simulink model "gm_HDL_pfc_gold_fi_vnl"  (R2024b)
settings: Solver=FixedStepDiscrete  StartTime=0.0  StopTime=.06  RelTol=1e-3
InitFcn:
  | fidelity_pfc_vals;
  | load('C:\Users\angro\Desktop\hil\pfc3ph\matlab\sim\sschdl\pfc_desktop\stateSpaceParameters.mat');
undefined symbols (not defined in the file or in its folder): a, b, c, DiscIntNeverNeededParam, fsw, Gs, s, stateSpaceParameters_1, t_ss, tsw
libraries: simulink x55, hdlmdlgenlib x26, hdlsllib x10, mcbcontrolslib x5, dspsrcs4 x3, slpidlib x2, hdlssclib x2, spsSVPWMGenerator2LevelLib x1, spsPLL3phLib x1
(part 2 of 4)

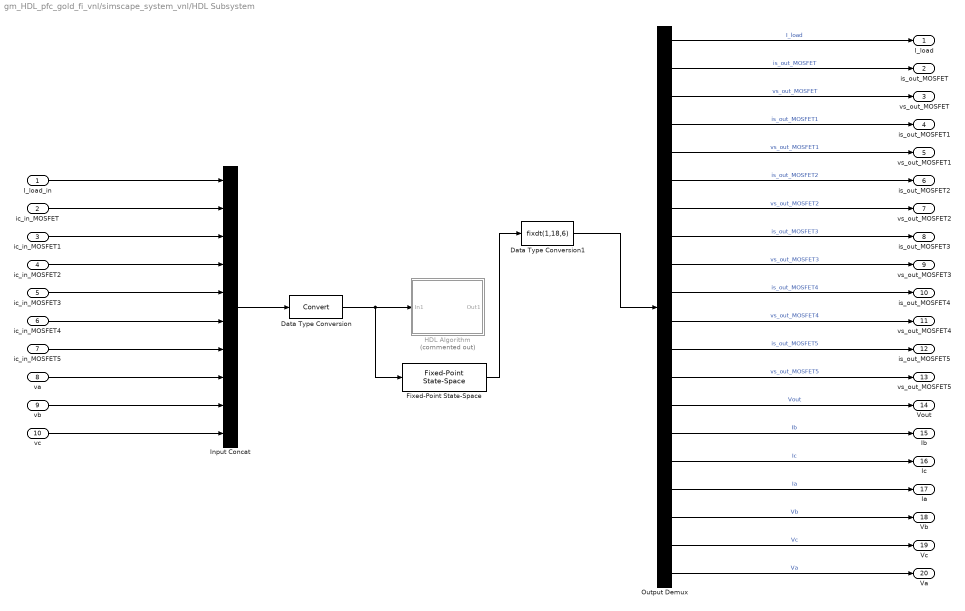
== system gm_HDL_pfc_gold_fi_vnl/simscape_system_vnl/HDL Subsystem ==
  I_load_in : Inport  OutDataTypeStr=fixdt(1,18,8)
  ic_in_MOSFET : Inport  Port=2  OutDataTypeStr=fixdt(1,18,8)
  ic_in_MOSFET1 : Inport  Port=3  OutDataTypeStr=fixdt(1,18,8)
  ic_in_MOSFET2 : Inport  Port=4  OutDataTypeStr=fixdt(1,18,8)
  ic_in_MOSFET3 : Inport  Port=5  OutDataTypeStr=fixdt(1,18,8)
  ic_in_MOSFET4 : Inport  Port=6  OutDataTypeStr=fixdt(1,18,8)
  ic_in_MOSFET5 : Inport  Port=7  OutDataTypeStr=fixdt(1,18,8)
  va : Inport  Port=8  OutDataTypeStr=fixdt(1,18,8)
  vb : Inport  Port=9  OutDataTypeStr=fixdt(1,18,8)
  vc : Inport  Port=10  OutDataTypeStr=fixdt(1,18,8)
  Data Type Conversion : DataTypeConversion  SaturateOnIntegerOverflow=off  RndMeth=Floor
  Data Type Conversion1 : DataTypeConversion  OutDataTypeStr=fixdt(1,18,6)  SaturateOnIntegerOverflow=off  RndMeth=Floor
  Fixed-Point State-Space : simulink/Additional Math & Discrete/Additional Discrete/Fixed-Point State-Space  A=fi(stateSpaceParameters_1.Ad,1,25,24)  B=fi(stateSpaceParameters_1.Bd,1,25,31)  C=fi(stateSpaceParameters_1.Cd,1,25,20)  D=fi(stateSpaceParameters_1.Dd,1,25,19)  InitialCondition=fi(stateSpaceParameters_1.X0,1,25,14)  InternalDataType=fixdt(1,25,13)  StateEqScaling=2^0  OutputEqScaling=2^0  DoSatur=off
  HDL Algorithm : Subsystem  Commented=on
  Input Concat : Concatenate  NumInputs=10
  Output Demux : Demux  Outputs=20
  I_load : Outport
  is_out_MOSFET : Outport  Port=2
  vs_out_MOSFET : Outport  Port=3
  is_out_MOSFET1 : Outport  Port=4
  vs_out_MOSFET1 : Outport  Port=5
  is_out_MOSFET2 : Outport  Port=6
  vs_out_MOSFET2 : Outport  Port=7
  is_out_MOSFET3 : Outport  Port=8
  vs_out_MOSFET3 : Outport  Port=9
  is_out_MOSFET4 : Outport  Port=10
  vs_out_MOSFET4 : Outport  Port=11
  is_out_MOSFET5 : Outport  Port=12
  vs_out_MOSFET5 : Outport  Port=13
  Vout : Outport  Port=14
  Ib : Outport  Port=15
  Ic : Outport  Port=16
  Ia : Outport  Port=17
  Vb : Outport  Port=18
  Vc : Outport  Port=19
  Va : Outport  Port=20
  wires:
  Fixed-Point State-Space/1 -> Data Type Conversion1/1
  Data Type Conversion/1 -> HDL Algorithm/1(In1), Fixed-Point State-Space/1
  Data Type Conversion1/1 -> Output Demux/1
  ic_in_MOSFET4/1 -> Input Concat/6
  va/1 -> Input Concat/8
  ic_in_MOSFET5/1 -> Input Concat/7
  ic_in_MOSFET2/1 -> Input Concat/4
  ic_in_MOSFET3/1 -> Input Concat/5
  I_load_in/1 -> Input Concat/1
  ic_in_MOSFET1/1 -> Input Concat/3
  vb/1 -> Input Concat/9
  Output Demux/20 -> Va/1  "Va"
  Output Demux/18 -> Vb/1  "Vb"
  Output Demux/19 -> Vc/1  "Vc"
  Output Demux/16 -> Ic/1  "Ic"
  Output Demux/14 -> Vout/1  "Vout"
  Output Demux/11 -> vs_out_MOSFET4/1  "vs_out_MOSFET4"
  Output Demux/9 -> vs_out_MOSFET3/1  "vs_out_MOSFET3"
  Output Demux/10 -> is_out_MOSFET4/1  "is_out_MOSFET4"
  Output Demux/12 -> is_out_MOSFET5/1  "is_out_MOSFET5"
  Output Demux/5 -> vs_out_MOSFET1/1  "vs_out_MOSFET1"
  Output Demux/13 -> vs_out_MOSFET5/1  "vs_out_MOSFET5"
  Output Demux/15 -> Ib/1  "Ib"
  Output Demux/8 -> is_out_MOSFET3/1  "is_out_MOSFET3"
  Output Demux/6 -> is_out_MOSFET2/1  "is_out_MOSFET2"
  vc/1 -> Input Concat/10
  Output Demux/1 -> I_load/1  "I_load"
  Output Demux/17 -> Ia/1  "Ia"
  Input Concat/1 -> Data Type Conversion/1
  ic_in_MOSFET/1 -> Input Concat/2
  Output Demux/4 -> is_out_MOSFET1/1  "is_out_MOSFET1"
  Output Demux/3 -> vs_out_MOSFET/1  "vs_out_MOSFET"
  Output Demux/2 -> is_out_MOSFET/1  "is_out_MOSFET"
  Output Demux/7 -> vs_out_MOSFET2/1  "vs_out_MOSFET2"

== system gm_HDL_pfc_gold_fi_vnl/Subsystem1/ctrl_pwm/PI_CTRL ==
  id : Inport
  iq : Inport  Port=2
  Add3 : Sum  Inputs=+-
  Add4 : Sum  Inputs=+-
  Constant : Constant  Value=0  SampleTime=t_ss
  Constant1 : Constant  Value=-6  SampleTime=t_ss
  Vd_ctrl : slpidlib/PID Controller  Controller=PI  Form=Parallel  TimeDomain=Discrete-time  UseExternalTs=off  SampleTime=t_ss  IntegratorMethod=Backward Euler  FilterMethod=Forward Euler  ControllerParametersSource=internal  P=-1.8  I=-.15  UseKiTs=off  D=0  UseExternalDerivativeSource=off  N=100  UseFilter=on  TunerSelectOption=Transfer Function Based (PID Tuner App)  InitialConditionSource=internal  InitialConditionForIntegrator=0  InitialConditionForFilter=0  DifferentiatorICPrevScaledInput=0  ExternalReset=none  TrackingMode=off  Kt=1  LimitOutput=off  SatLimitsSource=internal  UpperSaturationLimit=5e2  LowerSaturationLimit=-5e2  LinearizeAsGain=on  AntiWindupMode=clamping  Kb=1  LimitIntegrator=off  UpperIntegratorSaturationLimit=inf  LowerIntegratorSaturationLimit=-inf  POutMin=[]  POutMax=[]  IOutMin=[]  IOutMax=[]  DOutMin=[]  DOutMax=[]  NOutMin=[]  NOutMax=[]  SumOutMin=[]  SumOutMax=[]  SaturationOutMin=[]  SaturationOutMax=[]  PParamMin=[]  PParamMax=[]  IParamMin=[]  IParamMax=[]  DParamMin=[]  DParamMax=[]  NParamMin=[]  NParamMax=[]  KbParamMin=[]  KbParamMax=[]  KtParamMin=[]  KtParamMax=[]  KbOutMin=[]  KbOutMax=[]  KtOutMin=[]  KtOutMax=[]  IntegratorOutMin=[]  IntegratorOutMax=[]  FilterOutMin=[]  FilterOutMax=[]  SumI1OutMin=[]  SumI1OutMax=[]  SumI2OutMin=[]  SumI2OutMax=[]  SumI3OutMin=[]  SumI3OutMax=[]  SumI4OutMin=[]  SumI4OutMax=[]  SumDOutMin=[]  SumDOutMax=[]  DifferentiatorOutMin=[]  DifferentiatorOutMax=[]  FilterDiffOutCoefMin=[]  FilterDiffOutCoefMax=[]  ReciprocalOutMin=[]  ReciprocalOutMax=[]  SumDenOutMin=[]  SumDenOutMax=[]  SumNumOutMin=[]  SumNumOutMax=[]  DivideOutMin=[]  DivideOutMax=[]  UdiffTsProdOutMin=[]  UdiffTsProdOutMax=[]  NTsProdOutMin=[]  NTsProdOutMax=[]  UintegralTsProdOutMin=[]  UintegralTsProdOutMax=[]  UngainTsProdOutMin=[]  UngainTsProdOutMax=[]  ClampingZeroOutDataTypeStr=Inherit: Inherit via back propagation  ClampingZeroOutMin=[]  ClampingZeroOutMax=[]  FilterDenConstantOutDataTypeStr=Inherit: Inherit via back propagation  FilterDenConstantOutMin=[]  FilterDenConstantOutMax=[]  PCopyOutDataTypeStr=Inherit: Inherit via back propagation  PCopyOutMin=[]  PCopyOutMax=[]  NCopyOutDataTypeStr=Inherit: Inherit via back propagation  NCopyOutMin=[]  NCopyOutMax=[]  IntegratorContinuousStateAttributes=''  IntegratorStateMustResolveToSignalObject=off  IntegratorRTWStateStorageClass=Auto  FilterContinuousStateAttributes=''  FilterStateMustResolveToSignalObject=off  FilterRTWStateStorageClass=Auto  ParallelPVariant=InternalParameters  IdealPVariant=Disabled  IVariant=InternalParameters  DVariant=Disabled  IntegratorVariant=Discrete  SatVariant=Disabled  AWVariant=Passthrough  PCopyVariant=Disabled  TRVariant=Disabled  FdbkBlocksVariant=Forward  IdealPFdbkVariant=Disabled  SatFdbkVariant=Disabled  DerivativeFilterVariant=Disabled  NVariant=Disabled  NCopyVariant=Disabled_SignalSpec  FilterICVariant=Disabled  IntegratorICVariant=InternalICs  ExternalResetVariant=Disabled  TRSumVariant=Passthrough  SumFdbkVariant=Disabled  SumVariant=Sum_PI  TsampFilterVariant=InternalTs  TsampNgainVariant=Passthrough  TsampIntegralVariant=Disabled_SignalSpec  ExternalSaturationOutDataTypeStr=Inherit: Same as second input  DerivativeSourceVariant=Disabled  PreIntVariant=InternalPreInt
  Vq_ctrl : slpidlib/PID Controller  Controller=PI  Form=Parallel  TimeDomain=Discrete-time  UseExternalTs=off  SampleTime=t_ss  IntegratorMethod=Backward Euler  FilterMethod=Forward Euler  ControllerParametersSource=internal  P=-2  I=-.2  UseKiTs=off  D=0  UseExternalDerivativeSource=off  N=100  UseFilter=on  TunerSelectOption=Transfer Function Based (PID Tuner App)  InitialConditionSource=internal  InitialConditionForIntegrator=0  InitialConditionForFilter=0  DifferentiatorICPrevScaledInput=0  ExternalReset=none  TrackingMode=off  Kt=1  LimitOutput=off  SatLimitsSource=internal  UpperSaturationLimit=5e2  LowerSaturationLimit=-5e2  LinearizeAsGain=on  AntiWindupMode=clamping  Kb=1  LimitIntegrator=off  UpperIntegratorSaturationLimit=inf  LowerIntegratorSaturationLimit=-inf  POutMin=[]  POutMax=[]  IOutMin=[]  IOutMax=[]  DOutMin=[]  DOutMax=[]  NOutMin=[]  NOutMax=[]  SumOutMin=[]  SumOutMax=[]  SaturationOutMin=[]  SaturationOutMax=[]  PParamMin=[]  PParamMax=[]  IParamMin=[]  IParamMax=[]  DParamMin=[]  DParamMax=[]  NParamMin=[]  NParamMax=[]  KbParamMin=[]  KbParamMax=[]  KtParamMin=[]  KtParamMax=[]  KbOutMin=[]  KbOutMax=[]  KtOutMin=[]  KtOutMax=[]  IntegratorOutMin=[]  IntegratorOutMax=[]  FilterOutMin=[]  FilterOutMax=[]  SumI1OutMin=[]  SumI1OutMax=[]  SumI2OutMin=[]  SumI2OutMax=[]  SumI3OutMin=[]  SumI3OutMax=[]  SumI4OutMin=[]  SumI4OutMax=[]  SumDOutMin=[]  SumDOutMax=[]  DifferentiatorOutMin=[]  DifferentiatorOutMax=[]  FilterDiffOutCoefMin=[]  FilterDiffOutCoefMax=[]  ReciprocalOutMin=[]  ReciprocalOutMax=[]  SumDenOutMin=[]  SumDenOutMax=[]  SumNumOutMin=[]  SumNumOutMax=[]  DivideOutMin=[]  DivideOutMax=[]  UdiffTsProdOutMin=[]  UdiffTsProdOutMax=[]  NTsProdOutMin=[]  NTsProdOutMax=[]  UintegralTsProdOutMin=[]  UintegralTsProdOutMax=[]  UngainTsProdOutMin=[]  UngainTsProdOutMax=[]  ClampingZeroOutDataTypeStr=Inherit: Inherit via back propagation  ClampingZeroOutMin=[]  ClampingZeroOutMax=[]  FilterDenConstantOutDataTypeStr=Inherit: Inherit via back propagation  FilterDenConstantOutMin=[]  FilterDenConstantOutMax=[]  PCopyOutDataTypeStr=Inherit: Inherit via back propagation  PCopyOutMin=[]  PCopyOutMax=[]  NCopyOutDataTypeStr=Inherit: Inherit via back propagation  NCopyOutMin=[]  NCopyOutMax=[]  IntegratorContinuousStateAttributes=''  IntegratorStateMustResolveToSignalObject=off  IntegratorRTWStateStorageClass=Auto  FilterContinuousStateAttributes=''  FilterStateMustResolveToSignalObject=off  FilterRTWStateStorageClass=Auto  ParallelPVariant=InternalParameters  IdealPVariant=Disabled  IVariant=InternalParameters  DVariant=Disabled  IntegratorVariant=Discrete  SatVariant=Disabled  AWVariant=Passthrough  PCopyVariant=Disabled  TRVariant=Disabled  FdbkBlocksVariant=Forward  IdealPFdbkVariant=Disabled  SatFdbkVariant=Disabled  DerivativeFilterVariant=Disabled  NVariant=Disabled  NCopyVariant=Disabled_SignalSpec  FilterICVariant=Disabled  IntegratorICVariant=InternalICs  ExternalResetVariant=Disabled  TRSumVariant=Passthrough  SumFdbkVariant=Disabled  SumVariant=Sum_PI  TsampFilterVariant=InternalTs  TsampNgainVariant=Passthrough  TsampIntegralVariant=Disabled_SignalSpec  ExternalSaturationOutDataTypeStr=Inherit: Same as second input  DerivativeSourceVariant=Disabled  PreIntVariant=InternalPreInt
  Vd_inductor : Outport
  Vq_inductor : Outport  Port=2
  wires:
  Add3/1 -> Vd_ctrl/1  "error_id"
  id/1 -> Add3/2
  Constant/1 -> Add3/1
  iq/1 -> Add4/2
  Add4/1 -> Vq_ctrl/1  "error_iq"
  Vd_ctrl/1 -> Vd_inductor/1
  Vq_ctrl/1 -> Vq_inductor/1
  Constant1/1 -> Add4/1

== system gm_HDL_pfc_gold_fi_vnl/Subsystem1/ctrl_pwm/SVPWM ==
  Vd_inductor : Inport
  angle : Inport  Port=2
  Vq_inductor : Inport  Port=3
  Cos : Trigonometry  Operator=cos
  Inverse Park Transform : mcbcontrolslib/Inverse Park Transform  PhaseInput=Two inputs  AxisAlignment=D-axis  ThetaInput=Sine and Cosine electrical position  AngleInput=Per-unit  N_points=1024
  SVPWM Generator (2-Level) : spsSVPWMGenerator2LevelLib/SVPWM Generator (2-Level)  InputType=alpha-beta components  SwitchingPattern=Pattern #1  Fc=fsw*1e3  ParUref=[0.8 -30 50]  Ts=t_ss
  Sin : Trigonometry
  P : Outport
  wires:
  Vd_inductor/1 -> Inverse Park Transform/1
  Vq_inductor/1 -> Inverse Park Transform/2
  Inverse Park Transform/2 -> SVPWM Generator (2-Level)/2  "Vbet_indc"
  Sin/1 -> Inverse Park Transform/3
  Cos/1 -> Inverse Park Transform/4
  Inverse Park Transform/1 -> SVPWM Generator (2-Level)/1  "Valp_indc"
  angle/1 -> Cos/1, Sin/1
  SVPWM Generator (2-Level)/1 -> P/1

== system gm_HDL_pfc_gold_fi_vnl/Subsystem1/ctrl_pwm/transforms ==
  a : Inport
  b : Inport  Port=2
  In3 : Inport  Port=3
  In4 : Inport  Port=4
  In5 : Inport  Port=5
  Claro-Parl Transform : Subsystem  Commented=on
  Claro-Parl Transform1 : Subsystem
  Delay : Delay  DelayLength=1
  Delay1 : Delay  DelayLength=1
  Mux : Mux  Inputs=3
  PLL (3ph) : spsPLL3phLib/PLL (3ph)  Fmin=50  Par_Init=[0, 50]  ParK=[180,3200,1]  TcD=1e-4  MaxRateChangeFreq=12  FilterCutOffFreq=25  Ts=t_ss  AGC=on
  Terminator : Terminator
  id : Outport
  iq : Outport  Port=2
  angle : Outport  Port=3
  wires:
  Mux/1 -> PLL (3ph)/1
  PLL (3ph)/2 -> angle/1, Claro-Parl Transform1/3(wt), Claro-Parl Transform/3(wt)  "angle"
  PLL (3ph)/1 -> Terminator/1
  In3/1 -> Mux/1, Claro-Parl Transform/1(a)
  In5/1 -> Mux/3
  b/1 -> Delay1/1
  In4/1 -> Claro-Parl Transform/2(b), Mux/2
  a/1 -> Delay/1
  Delay/1 -> Claro-Parl Transform1/1(a)
  Delay1/1 -> Claro-Parl Transform1/2(b)
  Claro-Parl Transform/1(d) -> ?  "vd"
  Claro-Parl Transform/2(q) -> ?  "vq"
  Claro-Parl Transform1/1(d) -> id/1  "id"
  Claro-Parl Transform1/2(q) -> iq/1  "iq"

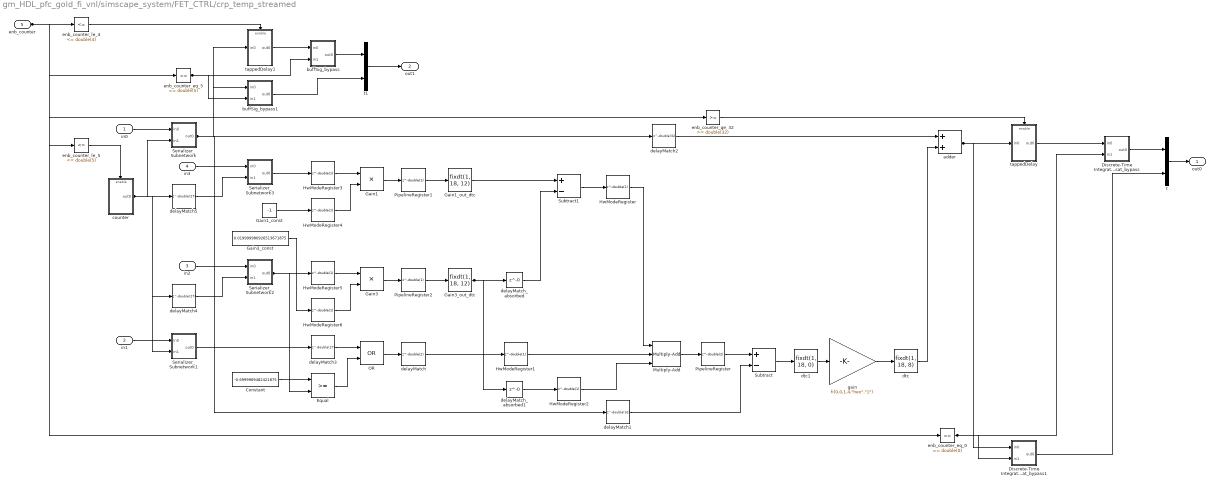
== system gm_HDL_pfc_gold_fi_vnl/simscape_system/FET_CTRL/crp_temp_streamed ==
  in0 : Inport  OutDataTypeStr=fixdt(1, 18, 8)  PortDimensions=[6]  SampleTime=1.38600138600139e-08
  in1 : Inport  Port=2  OutDataTypeStr=boolean  PortDimensions=[6]  SampleTime=1.38600138600139e-08
  in2 : Inport  Port=3  OutDataTypeStr=fixdt(1, 18, 6)  PortDimensions=[6]  SampleTime=1.38600138600139e-08
  in3 : Inport  Port=4  OutDataTypeStr=fixdt(1, 18, 6)  PortDimensions=[6]  SampleTime=1.38600138600139e-08
  enb_counter : Inport  Port=5  OutDataTypeStr=fixdt(0, 6, 0)  SampleTime=1.38600138600139e-08
  Constant : Constant  Value=-0.6999969482421875  OutDataTypeStr=fixdt(1, 18, 17)  SampleTime=1.38600138600139e-08
  Discrete-Time Integrator_u_sat_bypass : Subsystem
  Discrete-Time Integrator_u_sat_bypass1 : Subsystem
  Equal : RelationalOperator  OutDataTypeStr=boolean  SampleTime=1.38600138600139e-08  InputSameDT=off
  Gain1 : Product  Inputs=**  OutDataTypeStr=fixdt(1, 36, 23)  SampleTime=1.38600138600139e-08
  Gain1_const : Constant  Value=-1  OutDataTypeStr=fixdt(1, 18, 17)  SampleTime=1.38600138600139e-08
  Gain1_out_dtc : DataTypeConversion  OutDataTypeStr=fixdt(1, 18, 12)  SampleTime=1.38600138600139e-08  SaturateOnIntegerOverflow=off  RndMeth=Floor
  Gain3 : Product  Inputs=**  OutDataTypeStr=fixdt(1, 36, 28)  SampleTime=1.38600138600139e-08
  Gain3_const : Constant  Value=0.019999980926513671875  OutDataTypeStr=fixdt(1, 18, 22)  SampleTime=1.38600138600139e-08
  Gain3_out_dtc : DataTypeConversion  OutDataTypeStr=fixdt(1, 18, 12)  SampleTime=1.38600138600139e-08  SaturateOnIntegerOverflow=off  RndMeth=Floor
  HwModeRegister{,1..6} (7 alike) : Delay  DelayLength=double(1)  InitialCondition=0  SampleTime=1.38600138600139e-08
  Multiply-Add : hdlsllib/HDL Operations/Multiply-Add  Function=c+(a.*b)  datatype=fixdt(1, 18, 12)  DoSatur=off  FMA=off
  OR : Logic  Operator=OR  AllPortsSameDT=off  OutDataTypeStr=boolean  SampleTime=1.38600138600139e-08
  PipelineRegister : Delay  DelayLength=double(2)  InitialCondition=0  SampleTime=1.38600138600139e-08
  PipelineRegister1 : Delay  DelayLength=double(1)  InitialCondition=0  SampleTime=1.38600138600139e-08
  PipelineRegister2 : Delay  DelayLength=double(1)  InitialCondition=0  SampleTime=1.38600138600139e-08
  Serializer_Subnetwork : Subsystem
  Serializer_Subnetwork1 : Subsystem
  Serializer_Subnetwork2 : Subsystem
  Serializer_Subnetwork3 : Subsystem
  Subtract : Sum  Inputs=+-  OutDataTypeStr=fixdt(1, 18, 12)  AccumDataTypeStr=fixdt(1, 23, 12)  SampleTime=1.38600138600139e-08
  Subtract1 : Sum  Inputs=+-  OutDataTypeStr=fixdt(1, 18, 11)  AccumDataTypeStr=fixdt(1, 19, 12)  SampleTime=1.38600138600139e-08
  adder : Sum  OutDataTypeStr=fixdt(1, 18, 8)  AccumDataTypeStr=fixdt(1, 18, 8)  SampleTime=1.38600138600139e-08
  buffSig_bypass : Subsystem
  buffSig_bypass1 : Subsystem
  counter : Subsystem
  delayMatch : Delay  DelayLength=double(2)  InitialCondition=0  SampleTime=1.38600138600139e-08
  delayMatch1 : Delay  DelayLength=double(32)  InitialCondition=0  SampleTime=1.38600138600139e-08
  delayMatch2 : Delay  DelayLength=double(32)  InitialCondition=0  SampleTime=1.38600138600139e-08
  delayMatch3 : Delay  DelayLength=double(27)  InitialCondition=0  SampleTime=1.38600138600139e-08
  delayMatch4 : Delay  DelayLength=double(27)  InitialCondition=0  SampleTime=1.38600138600139e-08
  delayMatch5 : Delay  DelayLength=double(27)  InitialCondition=0  SampleTime=1.38600138600139e-08
  delayMatch_absorbed : Delay  DelayLength=0
  delayMatch_absorbed1 : Delay  DelayLength=0
  dtc : DataTypeConversion  OutDataTypeStr=fixdt(1, 18, 8)  ConvertRealWorld=Stored Integer (SI)  SampleTime=1.38600138600139e-08  SaturateOnIntegerOverflow=off  RndMeth=Floor
  dtc1 : DataTypeConversion  OutDataTypeStr=fixdt(1, 18, 0)  ConvertRealWorld=Stored Integer (SI)  SampleTime=1.38600138600139e-08  SaturateOnIntegerOverflow=off  RndMeth=Floor
  enb_counter_eq_0 : simulink/Logic and Bit Operations/Compare To Constant  relop===  const=double(0)  OutDataTypeStr=boolean
  enb_counter_eq_5 : simulink/Logic and Bit Operations/Compare To Constant  relop===  const=double(5)  OutDataTypeStr=boolean
  enb_counter_ge_32 : simulink/Logic and Bit Operations/Compare To Constant  relop=>=  const=double(32)  OutDataTypeStr=boolean
  enb_counter_le_4 : simulink/Logic and Bit Operations/Compare To Constant  relop=<=  const=double(4)  OutDataTypeStr=boolean
  enb_counter_le_5 : simulink/Logic and Bit Operations/Compare To Constant  relop=<=  const=double(5)  OutDataTypeStr=boolean
  gain : Gain  Gain="fi(0,0,1,4,\"hex\",\"1\")"  ParamDataTypeStr=fixdt(0, 1, 4)  OutDataTypeStr=fixdt(1, 18, 0)  SampleTime=1.38600138600139e-08
  t : Mux  Inputs=2
  t1 : Mux  Inputs=2
  tappedDelay : Subsystem
  tappedDelay1 : Subsystem
  out0 : Outport  OutDataTypeStr=fixdt(1, 18, 8)  PortDimensions=[6]  SampleTime=1.38600138600139e-08
  out1 : Outport  Port=2  OutDataTypeStr=fixdt(1, 18, 8)  PortDimensions=[6]  SampleTime=1.38600138600139e-08
  wires:
  Discrete-Time Integrator_u_sat_bypass/1(out0) -> t/1
  enb_counter_eq_0/1 -> Discrete-Time Integrator_u_sat_bypass1/2(in1), Discrete-Time Integrator_u_sat_bypass/2(in1)
  adder/1 -> Discrete-Time Integrator_u_sat_bypass1/1(in0), tappedDelay/1(in0)
  dtc/1 -> adder/2
  gain/1 -> dtc/1
  dtc1/1 -> gain/1
  Subtract/1 -> dtc1/1
  PipelineRegister/1 -> Subtract/1
  enb_counter_ge_32/1 -> tappedDelay/Enable
  Multiply-Add/1 -> PipelineRegister/1
  delayMatch1/1 -> Subtract/2
  delayMatch_absorbed1/1 -> HwModeRegister2/1
  delayMatch_absorbed/1 -> Subtract1/2
  Gain1_out_dtc/1 -> Subtract1/1
  PipelineRegister1/1 -> Gain1_out_dtc/1
  OR/1 -> delayMatch/1
  Gain3/1 -> PipelineRegister2/1
  Gain1/1 -> PipelineRegister1/1
  t1/1 -> out1/1
  delayMatch/1 -> HwModeRegister1/1
  Equal/1 -> OR/2
  HwModeRegister/1 -> Multiply-Add/1
  HwModeRegister6/1 -> Gain3/2
  HwModeRegister5/1 -> Gain3/1
  HwModeRegister4/1 -> Gain1/2
  HwModeRegister3/1 -> Gain1/1
  delayMatch3/1 -> OR/1
  Constant/1 -> Equal/1
  Gain3_out_dtc/1 -> delayMatch_absorbed1/1, delayMatch_absorbed/1
  Serializer_Subnetwork2/1(out0) -> HwModeRegister5/1, Equal/2
  Gain1_const/1 -> HwModeRegister4/1
  buffSig_bypass1/1(out0) -> t1/2
  tappedDelay1/1(out0) -> buffSig_bypass/1(in0)
  PipelineRegister2/1 -> Gain3_out_dtc/1
  delayMatch4/1 -> Serializer_Subnetwork2/2(in1)
  Discrete-Time Integrator_u_sat_bypass1/1(out0) -> t/2
  in2/1 -> Serializer_Subnetwork2/1(in0)
  delayMatch2/1 -> adder/1
  delayMatch5/1 -> Serializer_Subnetwork3/2(in1)
  HwModeRegister2/1 -> Multiply-Add/3
  in3/1 -> Serializer_Subnetwork3/1(in0)
  t/1 -> out0/1
  Serializer_Subnetwork/1(out0) -> buffSig_bypass1/1(in0), delayMatch1/1, delayMatch2/1, tappedDelay1/1(in0)
  in1/1 -> Serializer_Subnetwork1/1(in0)
  buffSig_bypass/1(out0) -> t1/1
  HwModeRegister1/1 -> Multiply-Add/2
  counter/1(out0) -> Serializer_Subnetwork/2(in1), Serializer_Subnetwork1/2(in1), delayMatch4/1, delayMatch5/1
  Serializer_Subnetwork3/1(out0) -> HwModeRegister3/1
  in0/1 -> Serializer_Subnetwork/1(in0)
  enb_counter_le_4/1 -> tappedDelay1/Enable
  enb_counter_le_5/1 -> counter/Enable
  Serializer_Subnetwork1/1(out0) -> delayMatch3/1
  Gain3_const/1 -> HwModeRegister6/1
  enb_counter_eq_5/1 -> buffSig_bypass1/2(in1), buffSig_bypass/2(in1)
  Subtract1/1 -> HwModeRegister/1
  enb_counter/1 -> enb_counter_le_4/1, enb_counter_le_5/1, enb_counter_eq_0/1, enb_counter_eq_5/1, enb_counter_ge_32/1
  tappedDelay/1(out0) -> Discrete-Time Integrator_u_sat_bypass/1(in0)

== system gm_HDL_pfc_gold_fi_vnl/simscape_system/HDL Subsystem/Sparse Matrix-Vector Product ==
  in0 : Inport  OutDataTypeStr=fixdt(1, 25, 13)  PortDimensions=[10]  SampleTime=1.38600138600139e-08
  selectSignal : Inport  Port=2  OutDataTypeStr=boolean  SampleTime=1.38600138600139e-08
  enb_counter : Inport  Port=3  OutDataTypeStr=fixdt(0, 6, 0)  SampleTime=1.38600138600139e-08
  SelectCols{1..6} (6 alike) : Selector  InputPortWidth=10  IndexOptions=Index vector (dialog)  Indices=double([2 3 4 5 6 7 8 9 10])  OutputSizes=double(1)
  SelectCols7 : Selector  InputPortWidth=10  IndexOptions=Index vector (dialog)  Indices=double([1 2 3 4 5 6 7 8 9])  OutputSizes=double(1)
  SelectRows1 : Selector  InputPortWidth=63  IndexOptions=Index vector (dialog)  Indices=double([2 9 16 23 30 37 44 51 58])  OutputSizes=double(1)
  SelectRows2 : Selector  InputPortWidth=63  IndexOptions=Index vector (dialog)  Indices=double([3 10 17 24 31 38 45 52 59])  OutputSizes=double(1)
  SelectRows3 : Selector  InputPortWidth=63  IndexOptions=Index vector (dialog)  Indices=double([4 11 18 25 32 39 46 53 60])  OutputSizes=double(1)
  SelectRows4 : Selector  InputPortWidth=63  IndexOptions=Index vector (dialog)  Indices=double([5 12 19 26 33 40 47 54 61])  OutputSizes=double(1)
  SelectRows5 : Selector  InputPortWidth=63  IndexOptions=Index vector (dialog)  Indices=double([6 13 20 27 34 41 48 55 62])  OutputSizes=double(1)
  SelectRows6 : Selector  InputPortWidth=63  IndexOptions=Index vector (dialog)  Indices=double([7 14 21 28 35 42 49 56 63])  OutputSizes=double(1)
  SelectRows7 : Selector  InputPortWidth=63  IndexOptions=Index vector (dialog)  Indices=double([1 8 15 22 29 36 43 50 57])  OutputSizes=double(1)
  concatenate : Concatenate  NumInputs=7
  configuration1_wire : hdlmdlgenlib/Buffer
  const : Constant  Value=[-0.000935040414333343505859375;0.00615119002759456634521484375;-0.003075595013797283172607421875;-0.003075595013797283172607421875;-0.003075600601732730865478515625;-0.003075600601732730865478515625;0.0061512016691267490386962890625;0.0004675202071666717529296875;-0.00615119002759456634521484375;0.003075595013797283172607421875;0.003075595013797283172607421875;0.003075600601732730865478515625;0.003075600601732730865478515625;-0.0061512016691267490386962890625;0.0004675202071666717529296875;0.003075595013797283172607421875;-0.00615119002759456634521484375;0.003075595013797283172607421875;-0.0061512016691267490386962890625;0.003075600601732730865478515625;0.003075600601732730865478515625;0.0004675202071666717529296875;0.003075595013797283172607421875;0.003075595013797283172607421875;-0.00615119002759456634521484375;0.003075600601732730865478515625;-0.0061512016691267490386962890625;0.003075600601732730865478515625;0.0004675202071666717529296875;-0.003075595013797283172607421875;0.00615119002759456634521484375;-0.003075595013797283172607421875;0.0061512016691267490386962890625;-0.003075600601732730865478515625;-0.003075600601732730865478515625;0.0004675202071666717529296875;-0.003075595013797283172607421875;-0.003075595013797283172607421875;0.00615119002759456634521484375;-0.003075600601732730865478515625;0.0061512016691267490386962890625;-0.003075600601732730865478515625;0.0004675202071666717529296875;0.0002460475079715251922607421875;-0.00012302398681640625;-0.00012302398681640625;-0.00012302398681640625;-0.00012302398681640625;0.0002460479736328125;0;-0.00012302398681640625;0.0002460475079715251922607421875;-0.00012302398681640625;0.0002460479736328125;-0.00012302398681640625;-0.00012302398681640625;0;-0.00012302398681640625;-0.00012302398681640625;0.0002460475079715251922607421875;-0.00012302398681640625;0.0002460479736328125;-0.00012302398681640625]  OutDataTypeStr=fixdt(1, 25, 31)  SampleTime=1.38600138600139e-08
  dtc{,1..6} (7 alike) : DataTypeConversion  OutDataTypeStr=fixdt(1, 25, 13)  RndMeth=Nearest  SampleTime=1.38600138600139e-08  SaturateOnIntegerOverflow=off
  hNNewMatrixB_shared : Subsystem
  terminator : Terminator
  matrixBOutSignal : Outport  OutDataTypeStr=fixdt(1, 25, 13)  PortDimensions=[7]  SampleTime=1.38600138600139e-08
  wires:
  concatenate/1 -> matrixBOutSignal/1
  dtc6/1 -> concatenate/7
  dtc5/1 -> concatenate/6
  dtc4/1 -> concatenate/5
  dtc3/1 -> concatenate/4
  dtc2/1 -> concatenate/3
  dtc1/1 -> concatenate/2
  dtc/1 -> concatenate/1
  hNNewMatrixB_shared/6(out5) -> dtc1/1
  hNNewMatrixB_shared/4(out3) -> dtc3/1
  hNNewMatrixB_shared/3(out2) -> dtc4/1
  hNNewMatrixB_shared/2(out1) -> dtc5/1
  hNNewMatrixB_shared/1(out0) -> dtc6/1
  enb_counter/1 -> hNNewMatrixB_shared/15(enb_counter)
  SelectCols1/1 -> hNNewMatrixB_shared/14(in13)
  SelectRows1/1 -> hNNewMatrixB_shared/13(in12)
  SelectCols2/1 -> hNNewMatrixB_shared/12(in11)
  SelectRows2/1 -> hNNewMatrixB_shared/11(in10)
  hNNewMatrixB_shared/5(out4) -> dtc2/1
  SelectCols3/1 -> hNNewMatrixB_shared/10(in9)
  SelectRows3/1 -> hNNewMatrixB_shared/9(in8)
  SelectCols4/1 -> hNNewMatrixB_shared/8(in7)
  SelectRows4/1 -> hNNewMatrixB_shared/7(in6)
  hNNewMatrixB_shared/7(out6) -> dtc/1
  SelectCols5/1 -> hNNewMatrixB_shared/6(in5)
  SelectRows5/1 -> hNNewMatrixB_shared/5(in4)
  SelectCols6/1 -> hNNewMatrixB_shared/4(in3)
  SelectRows6/1 -> hNNewMatrixB_shared/3(in2)
  in0/1 -> SelectCols1/1, SelectCols5/1, SelectCols4/1, SelectCols2/1, SelectCols3/1, SelectCols7/1, SelectCols6/1
  SelectCols7/1 -> hNNewMatrixB_shared/2(in1)
  const/1 -> configuration1_wire/1
  SelectRows7/1 -> hNNewMatrixB_shared/1(in0)
  selectSignal/1 -> terminator/1
  configuration1_wire/1 -> SelectRows1/1, SelectRows3/1, SelectRows2/1, SelectRows4/1, SelectRows7/1, SelectRows5/1, SelectRows6/1

== system gm_HDL_pfc_gold_fi_vnl/simscape_system/HDL Subsystem/Sparse Matrix-Vector Product1 ==
  delayOutSignal : Inport  OutDataTypeStr=fixdt(1, 25, 13)  PortDimensions=[7]  SampleTime=1.38600138600139e-08
  selectSignal : Inport  Port=2  OutDataTypeStr=boolean  SampleTime=1.38600138600139e-08
  enb_counter : Inport  Port=3  OutDataTypeStr=fixdt(0, 6, 0)  SampleTime=1.38600138600139e-08
  SelectCols{1..6} (6 alike) : Selector  InputPortWidth=7  IndexOptions=Index vector (dialog)  Indices=double([1 2 3 4 5 6])  OutputSizes=double(1)
  SelectCols7 : Selector  InputPortWidth=7  IndexOptions=Index vector (dialog)  Indices=double([1 2 3 4 5 7])  OutputSizes=double(1)
  SelectRows1 : Selector  InputPortWidth=42  IndexOptions=Index vector (dialog)  Indices=double([1 8 15 22 29 36])  OutputSizes=double(1)
  SelectRows2 : Selector  InputPortWidth=42  IndexOptions=Index vector (dialog)  Indices=double([2 9 16 23 30 37])  OutputSizes=double(1)
  SelectRows3 : Selector  InputPortWidth=42  IndexOptions=Index vector (dialog)  Indices=double([3 10 17 24 31 38])  OutputSizes=double(1)
  SelectRows4 : Selector  InputPortWidth=42  IndexOptions=Index vector (dialog)  Indices=double([4 11 18 25 32 39])  OutputSizes=double(1)
  SelectRows5 : Selector  InputPortWidth=42  IndexOptions=Index vector (dialog)  Indices=double([5 12 19 26 33 40])  OutputSizes=double(1)
  SelectRows6 : Selector  InputPortWidth=42  IndexOptions=Index vector (dialog)  Indices=double([6 13 20 27 34 41])  OutputSizes=double(1)
  SelectRows7 : Selector  InputPortWidth=42  IndexOptions=Index vector (dialog)  Indices=double([7 14 21 28 35 42])  OutputSizes=double(1)
  concatenate : Concatenate  NumInputs=7
  configuration1_wire : hdlmdlgenlib/Buffer
  const : Constant  Value=[0.559759318828582763671875;-0.27987849712371826171875;-0.27987849712371826171875;-0.279879033565521240234375;-0.279879033565521240234375;0.55975806713104248046875;0;-0.27987849712371826171875;0.559759318828582763671875;-0.27987849712371826171875;0.55975806713104248046875;-0.279879033565521240234375;-0.279879033565521240234375;0;-0.27987849712371826171875;-0.27987849712371826171875;0.559759318828582763671875;-0.279879033565521240234375;0.55975806713104248046875;-0.279879033565521240234375;0;-0.05037820339202880859375;0.100756466388702392578125;-0.05037820339202880859375;0.100757062435150146484375;-0.050378322601318359375;-0.050378322601318359375;0;-0.05037820339202880859375;-0.05037820339202880859375;0.100756466388702392578125;-0.050378322601318359375;0.100757062435150146484375;-0.050378322601318359375;0;0.100756466388702392578125;-0.05037820339202880859375;-0.05037820339202880859375;-0.050378322601318359375;-0.050378322601318359375;0.100757062435150146484375;0.999971926212310791015625]  OutDataTypeStr=fixdt(1, 25, 24)  SampleTime=1.38600138600139e-08
  dtc{,1..6} (7 alike) : DataTypeConversion  OutDataTypeStr=fixdt(1, 25, 13)  RndMeth=Nearest  SampleTime=1.38600138600139e-08  SaturateOnIntegerOverflow=off
  hNNewMatrixA_shared : Subsystem
  terminator : Terminator
  matrixAOutSignal : Outport  OutDataTypeStr=fixdt(1, 25, 13)  PortDimensions=[7]  SampleTime=1.38600138600139e-08
  wires:
  concatenate/1 -> matrixAOutSignal/1
  dtc6/1 -> concatenate/7
  dtc5/1 -> concatenate/6
  dtc4/1 -> concatenate/5
  dtc3/1 -> concatenate/4
  dtc2/1 -> concatenate/3
  dtc1/1 -> concatenate/2
  dtc/1 -> concatenate/1
  hNNewMatrixA_shared/7(out6) -> dtc/1
  hNNewMatrixA_shared/5(out4) -> dtc2/1
  hNNewMatrixA_shared/4(out3) -> dtc3/1
  hNNewMatrixA_shared/3(out2) -> dtc4/1
  hNNewMatrixA_shared/2(out1) -> dtc5/1
  hNNewMatrixA_shared/1(out0) -> dtc6/1
  SelectCols1/1 -> hNNewMatrixA_shared/14(in13)
  SelectRows1/1 -> hNNewMatrixA_shared/13(in12)
  SelectCols2/1 -> hNNewMatrixA_shared/12(in11)
  SelectRows2/1 -> hNNewMatrixA_shared/11(in10)
  hNNewMatrixA_shared/6(out5) -> dtc1/1
  SelectCols3/1 -> hNNewMatrixA_shared/10(in9)
  SelectRows3/1 -> hNNewMatrixA_shared/9(in8)
  SelectCols4/1 -> hNNewMatrixA_shared/8(in7)
  SelectRows4/1 -> hNNewMatrixA_shared/7(in6)
  SelectCols5/1 -> hNNewMatrixA_shared/6(in5)
  enb_counter/1 -> hNNewMatrixA_shared/15(enb_counter)
  SelectRows5/1 -> hNNewMatrixA_shared/5(in4)
  SelectCols6/1 -> hNNewMatrixA_shared/4(in3)
  SelectCols7/1 -> hNNewMatrixA_shared/2(in1)
  SelectRows7/1 -> hNNewMatrixA_shared/1(in0)
  delayOutSignal/1 -> SelectCols7/1, SelectCols1/1, SelectCols6/1, SelectCols4/1, SelectCols2/1, SelectCols3/1, SelectCols5/1
  const/1 -> configuration1_wire/1
  configuration1_wire/1 -> SelectRows1/1, SelectRows6/1, SelectRows2/1, SelectRows3/1, SelectRows5/1, SelectRows4/1, SelectRows7/1
  SelectRows6/1 -> hNNewMatrixA_shared/3(in2)
  selectSignal/1 -> terminator/1

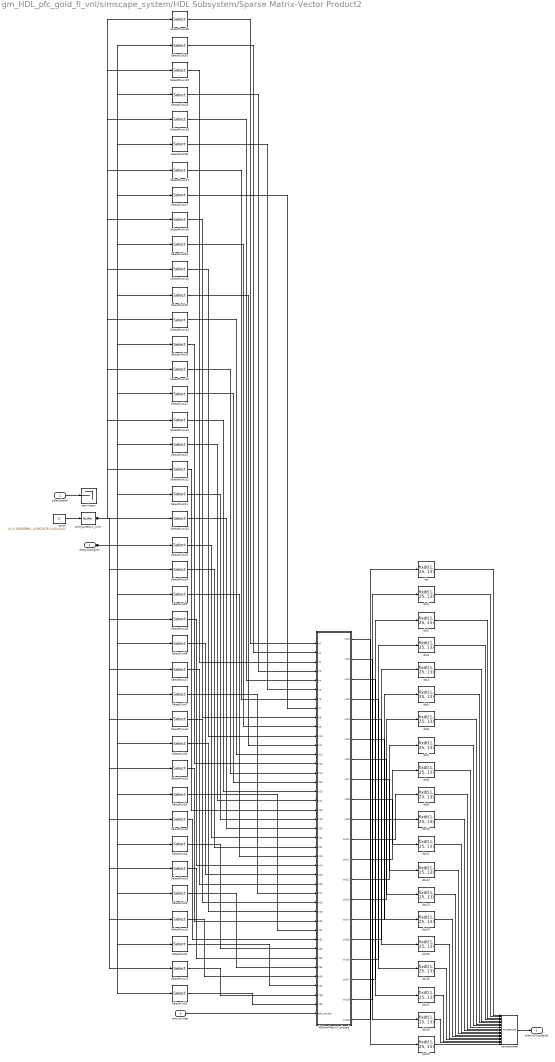
== system gm_HDL_pfc_gold_fi_vnl/simscape_system/HDL Subsystem/Sparse Matrix-Vector Product2 ==
  delayOutSignal : Inport  OutDataTypeStr=fixdt(1, 25, 13)  PortDimensions=[7]  SampleTime=1.38600138600139e-08
  selectSignal : Inport  Port=2  OutDataTypeStr=boolean  SampleTime=1.38600138600139e-08
  enb_counter : Inport  Port=3  OutDataTypeStr=fixdt(0, 6, 0)  SampleTime=1.38600138600139e-08
  SelectCols{1..20} (20 alike) : Selector  InputPortWidth=7  IndexOptions=Index vector (dialog)  Indices=double([1 2 3 4 5 6 7])  OutputSizes=double(1)
  SelectRows1 : Selector  InputPortWidth=140  IndexOptions=Index vector (dialog)  Indices=double([1 21 41 61 81 101 121])  OutputSizes=double(1)
  SelectRows10 : Selector  InputPortWidth=140  IndexOptions=Index vector (dialog)  Indices=double([10 30 50 70 90 110 130])  OutputSizes=double(1)
  SelectRows11 : Selector  InputPortWidth=140  IndexOptions=Index vector (dialog)  Indices=double([11 31 51 71 91 111 131])  OutputSizes=double(1)
  SelectRows12 : Selector  InputPortWidth=140  IndexOptions=Index vector (dialog)  Indices=double([12 32 52 72 92 112 132])  OutputSizes=double(1)
  SelectRows13 : Selector  InputPortWidth=140  IndexOptions=Index vector (dialog)  Indices=double([13 33 53 73 93 113 133])  OutputSizes=double(1)
  SelectRows14 : Selector  InputPortWidth=140  IndexOptions=Index vector (dialog)  Indices=double([14 34 54 74 94 114 134])  OutputSizes=double(1)
  SelectRows15 : Selector  InputPortWidth=140  IndexOptions=Index vector (dialog)  Indices=double([15 35 55 75 95 115 135])  OutputSizes=double(1)
  SelectRows16 : Selector  InputPortWidth=140  IndexOptions=Index vector (dialog)  Indices=double([16 36 56 76 96 116 136])  OutputSizes=double(1)
  SelectRows17 : Selector  InputPortWidth=140  IndexOptions=Index vector (dialog)  Indices=double([17 37 57 77 97 117 137])  OutputSizes=double(1)
  SelectRows18 : Selector  InputPortWidth=140  IndexOptions=Index vector (dialog)  Indices=double([18 38 58 78 98 118 138])  OutputSizes=double(1)
  SelectRows19 : Selector  InputPortWidth=140  IndexOptions=Index vector (dialog)  Indices=double([19 39 59 79 99 119 139])  OutputSizes=double(1)
  SelectRows2 : Selector  InputPortWidth=140  IndexOptions=Index vector (dialog)  Indices=double([2 22 42 62 82 102 122])  OutputSizes=double(1)
  SelectRows20 : Selector  InputPortWidth=140  IndexOptions=Index vector (dialog)  Indices=double([20 40 60 80 100 120 140])  OutputSizes=double(1)
  SelectRows3 : Selector  InputPortWidth=140  IndexOptions=Index vector (dialog)  Indices=double([3 23 43 63 83 103 123])  OutputSizes=double(1)
  SelectRows4 : Selector  InputPortWidth=140  IndexOptions=Index vector (dialog)  Indices=double([4 24 44 64 84 104 124])  OutputSizes=double(1)
  SelectRows5 : Selector  InputPortWidth=140  IndexOptions=Index vector (dialog)  Indices=double([5 25 45 65 85 105 125])  OutputSizes=double(1)
  SelectRows6 : Selector  InputPortWidth=140  IndexOptions=Index vector (dialog)  Indices=double([6 26 46 66 86 106 126])  OutputSizes=double(1)
  SelectRows7 : Selector  InputPortWidth=140  IndexOptions=Index vector (dialog)  Indices=double([7 27 47 67 87 107 127])  OutputSizes=double(1)
  SelectRows8 : Selector  InputPortWidth=140  IndexOptions=Index vector (dialog)  Indices=double([8 28 48 68 88 108 128])  OutputSizes=double(1)
  SelectRows9 : Selector  InputPortWidth=140  IndexOptions=Index vector (dialog)  Indices=double([9 29 49 69 89 109 129])  OutputSizes=double(1)
  concatenate : Concatenate  NumInputs=20
  configuration1_wire : hdlmdlgenlib/Buffer
  const : Constant  Value=[0;-0.16666698455810546875;-8.33333301544189453125;0.16666698455810546875;8.33333301544189453125;-0.08333301544189453125;-4.1666660308837890625;-0.08333301544189453125;-4.16666698455810546875;0.08333301544189453125;4.16666698455810546875;0.08333301544189453125;4.16666698455810546875;0;-0.16666698455810546875;-0.16666698455810546875;0.33333301544189453125;0;0;0;0;0.08333301544189453125;4.16666698455810546875;-0.08333301544189453125;-4.1666660308837890625;0.16666698455810546875;8.33333301544189453125;-0.08333301544189453125;-4.16666698455810546875;-0.16666698455810546875;-8.33333301544189453125;0.08333301544189453125;4.16666698455810546875;0;0.33333301544189453125;-0.16666698455810546875;-0.16666698455810546875;0;0;0;0;0.08333301544189453125;4.16666698455810546875;-0.08333301544189453125;-4.16666698455810546875;-0.08333301544189453125;-4.16666698455810546875;0.16666698455810546875;8.33333301544189453125;0.08333301544189453125;4.16666698455810546875;-0.16666698455810546875;-8.33333301544189453125;0;-0.16666698455810546875;0.33333301544189453125;-0.16666698455810546875;0;0;0;0;0.08333301544189453125;4.16666698455810546875;-0.08333301544189453125;-4.1666660308837890625;0.16666698455810546875;8.33333301544189453125;-0.08333301544189453125;-4.16666698455810546875;-0.16666698455810546875;-8.33333301544189453125;0.08333301544189453125;4.16666698455810546875;0;0.33333301544189453125;-0.16666698455810546875;-0.16666698455810546875;0;0;0;0;0.08333301544189453125;4.16666698455810546875;-0.08333301544189453125;-4.16666698455810546875;-0.08333301544189453125;-4.16666698455810546875;0.16666698455810546875;8.33333301544189453125;0.08333301544189453125;4.16666698455810546875;-0.16666698455810546875;-8.33333301544189453125;0;-0.16666698455810546875;0.33333301544189453125;-0.16666698455810546875;0;0;0;0;-0.16666698455810546875;-8.33333301544189453125;0.16666698455810546875;8.33333301544189453125;-0.08333301544189453125;-4.16666698455810546875;-0.08333301544189453125;-4.16666698455810546875;0.08333301544189453125;4.16666698455810546875;0.08333301544189453125;4.16666698455810546875;0;-0.16666698455810546875;-0.16666698455810546875;0.33333301544189453125;0;0;0;0;0.009998321533203125;0.4999103546142578125;0.009998321533203125;0.4999103546142578125;0.009998321533203125;0.4999103546142578125;0.009998321533203125;0.4999103546142578125;0.009998321533203125;0.4999103546142578125;0.009998321533203125;0.4999103546142578125;0.99981975555419921875;0;0;0;0;0;0]  OutDataTypeStr=fixdt(1, 25, 20)  SampleTime=1.38600138600139e-08
  dtc{,1..19} (20 alike) : DataTypeConversion  OutDataTypeStr=fixdt(1, 25, 13)  RndMeth=Nearest  SampleTime=1.38600138600139e-08  SaturateOnIntegerOverflow=off
  hNNewMatrixC_shared : Subsystem
  terminator : Terminator
  matrixCOutSignal : Outport  OutDataTypeStr=fixdt(1, 25, 13)  PortDimensions=[20]  SampleTime=1.38600138600139e-08
  wires:
  concatenate/1 -> matrixCOutSignal/1
  dtc19/1 -> concatenate/20
  dtc18/1 -> concatenate/19
  dtc17/1 -> concatenate/18
  dtc16/1 -> concatenate/17
  dtc15/1 -> concatenate/16
  dtc14/1 -> concatenate/15
  dtc13/1 -> concatenate/14
  dtc12/1 -> concatenate/13
  dtc11/1 -> concatenate/12
  dtc10/1 -> concatenate/11
  dtc9/1 -> concatenate/10
  dtc8/1 -> concatenate/9
  dtc7/1 -> concatenate/8
  dtc6/1 -> concatenate/7
  dtc5/1 -> concatenate/6
  dtc4/1 -> concatenate/5
  dtc3/1 -> concatenate/4
  dtc2/1 -> concatenate/3
  dtc1/1 -> concatenate/2
  dtc/1 -> concatenate/1
  hNNewMatrixC_shared/20(out19) -> dtc/1
  hNNewMatrixC_shared/16(out15) -> dtc4/1
  hNNewMatrixC_shared/13(out12) -> dtc7/1
  hNNewMatrixC_shared/7(out6) -> dtc13/1
  hNNewMatrixC_shared/6(out5) -> dtc14/1
  hNNewMatrixC_shared/4(out3) -> dtc16/1
  hNNewMatrixC_shared/3(out2) -> dtc17/1
  enb_counter/1 -> hNNewMatrixC_shared/41(enb_counter)
  SelectCols1/1 -> hNNewMatrixC_shared/40(in39)
  hNNewMatrixC_shared/5(out4) -> dtc15/1
  SelectCols2/1 -> hNNewMatrixC_shared/38(in37)
  hNNewMatrixC_shared/1(out0) -> dtc19/1
  SelectCols3/1 -> hNNewMatrixC_shared/36(in35)
  SelectCols4/1 -> hNNewMatrixC_shared/34(in33)
  SelectRows4/1 -> hNNewMatrixC_shared/33(in32)
  SelectCols5/1 -> hNNewMatrixC_shared/32(in31)
  hNNewMatrixC_shared/14(out13) -> dtc6/1
  SelectCols6/1 -> hNNewMatrixC_shared/30(in29)
  SelectRows3/1 -> hNNewMatrixC_shared/35(in34)
  hNNewMatrixC_shared/10(out9) -> dtc10/1
  SelectRows6/1 -> hNNewMatrixC_shared/29(in28)
  hNNewMatrixC_shared/9(out8) -> dtc11/1
  hNNewMatrixC_shared/12(out11) -> dtc8/1
  SelectCols7/1 -> hNNewMatrixC_shared/28(in27)
  SelectCols8/1 -> hNNewMatrixC_shared/26(in25)
  hNNewMatrixC_shared/19(out18) -> dtc1/1
  SelectRows8/1 -> hNNewMatrixC_shared/25(in24)
  SelectCols9/1 -> hNNewMatrixC_shared/24(in23)
  SelectRows9/1 -> hNNewMatrixC_shared/23(in22)
  SelectCols10/1 -> hNNewMatrixC_shared/22(in21)
  SelectRows10/1 -> hNNewMatrixC_shared/21(in20)
  SelectCols11/1 -> hNNewMatrixC_shared/20(in19)
  SelectRows7/1 -> hNNewMatrixC_shared/27(in26)
  SelectRows11/1 -> hNNewMatrixC_shared/19(in18)
  SelectCols12/1 -> hNNewMatrixC_shared/18(in17)
  SelectRows12/1 -> hNNewMatrixC_shared/17(in16)
  SelectCols13/1 -> hNNewMatrixC_shared/16(in15)
  SelectRows13/1 -> hNNewMatrixC_shared/15(in14)
  hNNewMatrixC_shared/18(out17) -> dtc2/1
  SelectRows5/1 -> hNNewMatrixC_shared/31(in30)
  SelectCols14/1 -> hNNewMatrixC_shared/14(in13)
  SelectCols15/1 -> hNNewMatrixC_shared/12(in11)
  SelectRows15/1 -> hNNewMatrixC_shared/11(in10)
  SelectCols16/1 -> hNNewMatrixC_shared/10(in9)
  SelectRows16/1 -> hNNewMatrixC_shared/9(in8)
  SelectRows1/1 -> hNNewMatrixC_shared/39(in38)
  SelectCols17/1 -> hNNewMatrixC_shared/8(in7)
  SelectCols18/1 -> hNNewMatrixC_shared/6(in5)
  SelectRows18/1 -> hNNewMatrixC_shared/5(in4)
  hNNewMatrixC_shared/2(out1) -> dtc18/1
  hNNewMatrixC_shared/8(out7) -> dtc12/1
  SelectCols19/1 -> hNNewMatrixC_shared/4(in3)
  SelectCols20/1 -> hNNewMatrixC_shared/2(in1)
  SelectRows19/1 -> hNNewMatrixC_shared/3(in2)
  hNNewMatrixC_shared/15(out14) -> dtc5/1
  hNNewMatrixC_shared/11(out10) -> dtc9/1
  SelectRows20/1 -> hNNewMatrixC_shared/1(in0)
  delayOutSignal/1 -> SelectCols8/1, SelectCols6/1, SelectCols1/1, SelectCols7/1, SelectCols2/1, SelectCols4/1, SelectCols3/1, SelectCols13/1, SelectCols5/1, SelectCols9/1, SelectCols10/1, SelectCols11/1, SelectCols12/1, SelectCols14/1, SelectCols15/1, SelectCols16/1, SelectCols17/1, SelectCols18/1, SelectCols19/1, SelectCols20/1
  const/1 -> configuration1_wire/1
  SelectRows14/1 -> hNNewMatrixC_shared/13(in12)
  selectSignal/1 -> terminator/1
  configuration1_wire/1 -> SelectRows1/1, SelectRows6/1, SelectRows2/1, SelectRows3/1, SelectRows5/1, SelectRows15/1, SelectRows4/1, SelectRows7/1, SelectRows8/1, SelectRows9/1, SelectRows10/1, SelectRows11/1, SelectRows12/1, SelectRows13/1, SelectRows14/1, SelectRows16/1, SelectRows17/1, SelectRows19/1, SelectRows18/1, SelectRows20/1
  SelectRows17/1 -> hNNewMatrixC_shared/7(in6)
  hNNewMatrixC_shared/17(out16) -> dtc3/1
  SelectRows2/1 -> hNNewMatrixC_shared/37(in36)
